simulink model "lorenz_attractor"  (R2025b)
settings: Solver=ode23  StartTime=0  StopTime=100  RelTol=1e-3
StopFcn:
  | LorenzAttraktorStopFcn
settings Model: Creator=danieltchoudovski  LastModifiedBy=danieltchoudovski
settings DataIOCC: SaveFormat=Array  SaveState=on  TimeSaveName=t

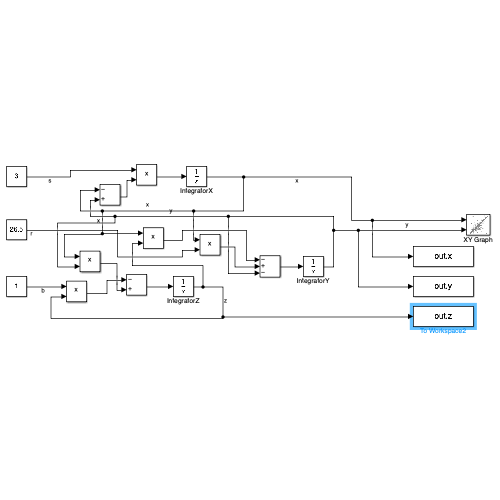
[thumbnail: Simulink's stored preview of the top-level diagram]
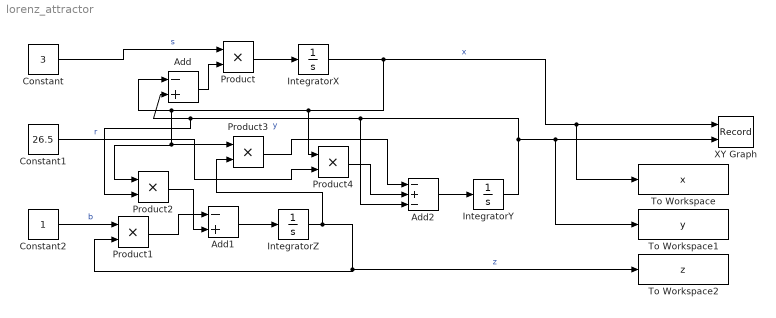
== system lorenz_attractor ==
  Add : Sum  Inputs=-+
  Add1 : Sum  Inputs=-+
  Add2 : Sum  Inputs=-+-
  Constant : Constant  Value=3
  Constant1 : Constant  Value=26.5
  Constant2 : Constant
  IntegratorX : Integrator  InitialCondition=5
  IntegratorY : Integrator  InitialCondition=5
  IntegratorZ : Integrator  InitialCondition=5
  Product{,1..4} (5 alike) : Product
  To Workspace : ToWorkspace  VariableName=x  SaveFormat=Timeseries  SampleTime=-1
  To Workspace1 : ToWorkspace  VariableName=y  SaveFormat=Timeseries  SampleTime=-1
  To Workspace2 : ToWorkspace  VariableName=z  SaveFormat=Timeseries  SampleTime=-1
  XY Graph : Record  NumPorts=2.0  FileSettingsInternal="{\"entries\":[{\"content\":{\"excelSettings\":{\"content\":{},\"type\":\"Streamout.ExcelSettings\"},\"parquetSettings\":{\"content\":{},\"type\":\"Streamout.ParquetSettings\"}},\"type\":\"Streamout.FileSettingStorage\",\"uuid\":\"\"}],\"packageUris\":[\"http:\\/\\/schema.mathworks.com\\/mf0\\/streamout_blocks\\/R2020a\"],\"version\":\"1.0\"}"  FrameSettings=[0, 0]  Layout=[1 1]  SignalsInternal="{\"entries\":[{\"content\":{\"signals\":[{\"content\":{\"blockPath\":[],\"dimensions\":[1],\"domain\":\"\",\"lineColor\":\"#64d413\",\"lineWidth\":2,\"port\":1,\"sid\":[\"\"],\"signalID\":1,\"signalName\":\"x\"},\"type\":\"RecordBlkView.Signal\",\"uuid\":\"\"},{\"content\":{\"blockPath\":[],\"dimensions\":[1],\"domain\":\"\",\"lineColor\":\"#ff13a6\",\"lineWidth\":2,\"port\":2,\"sid\":[\"\"],\"signalID\":2,\"signalName\":\"y\"},\"type\":\"RecordBlkView.Signal\",\"uuid\":\"\"}]},\"type\":\"RecordBlkView.InputSignals\",\"uuid\":\"\"}],\"packageUris\":[\"http:\\/\\/schema.mathworks.com\\/mf0\\/streamout_blocks\\/R2020a\"],\"version\":\"1.0\"}"  VisualizationBindings="{\"xyplotplugin\":{\"info\":[{\"series\":[{\"bindingParametersList\":[{\"parameter\":\"X-Axis\",\"signalID\":233,\"signalName\":\"x\"},{\"parameter\":\"Y-Axis\",\"signalID\":237,\"signalName\":\"y\"}],\"seriesID\":0}],\"subplotID\":1}]}}"  CompatibilityTag=XY
  wires:
  IntegratorX/1 -> Product4/1, Product3/1, Product2/1, Add/1, To Workspace/1, XY Graph/1  "x"
  IntegratorY/1 -> Product2/2, Add/2, Add2/3, To Workspace1/1, XY Graph/2  "y"
  IntegratorZ/1 -> Product3/2, To Workspace2/1, Product1/2  "z"
  Constant/1 -> Product/1  "s"
  Constant1/1 -> Product4/2  "r"
  Constant2/1 -> Product1/1  "b"
  Product/1 -> IntegratorX/1
  Add/1 -> Product/2
  Add1/1 -> IntegratorZ/1
  Product1/1 -> Add1/1
  Product2/1 -> Add1/2
  Product3/1 -> Add2/1
  Add2/1 -> IntegratorY/1
  Product4/1 -> Add2/2
